simulink model "DC_AC"  (R2023a)
settings: Solver=VariableStepAuto  StartTime=0.0  StopTime=1.5  MaxStep=1e-4  RelTol=1e-3
libraries: spsMosfetLib x32, spsSeriesRLCBranchLib x29, simulink x25, spsCurrentMeasurementLib x11, spsVoltageMeasurementLib x9, spsDCVoltageSourceLib x8, spsIdealSwitchLib x5, spsDiodeLib x1, spspowerguiLib x1
(part 2 of 2)

== matlab function DC_AC/MATLAB Function ==
  data: flag input; Q14 output; compare_data input; Q23 output; u input
function [Q14,Q23]= fcn(flag, compare_data, u)

if flag == 1 %说明在正半周
    if u > compare_data %Q14导通
        Q14 = 1;        %在高电平阶段
        Q23 = 0;
    else
        Q14 = 0;
        Q23 = 0;
    end
else      %说明在负半周
    if u > compare_data
        Q23 = 1;
        Q14 = 0;
    else
        Q23 = 0;
        Q14 = 0;
    end
end

== matlab function DC_AC/Cϕx_Calculation1 ==
  data: x_Matrix input; y output; Phi input; c_Matrix input
function y = fcn(x_Matrix,Phi,c_Matrix)
a = x_Matrix;
b = Phi;
c = transpose(c_Matrix);
d = c*b
y = c*b*a;

== matlab function DC_AC/Distrubance_Calculation2 ==
  data: u input; D1_K_1 output; D1_K_2 output; D2_K_1 output; D2_K_2 output
function [D1_K_1,D1_K_2,D2_K_1,D2_K_2] = fcn(u)
d1_k_1 = (u(3)-u(4))/u(5)-u(2);
d2_k_1 = (u(1)-u(2)/u(5))-(u(6)*u(11)/(u(7)*u(8)))-(u(4)/(u(7)*u(8)))-(u(10)/(u(7)*u(8)))-(u(2)/(u(9)*u(8)));%d2(k-1)


D1_K_1 = d1_k_1;
D2_K_1 = d2_k_1;
D1_K_2 = u(12);
D2_K_2 = u(13);

== matlab function DC_AC/Distrubance_Calculation3 ==
  data: D1_K_1 input; C_d_Value output; D1_K_2 input; D2_K_1 input; D2_K_2 input; c input
function C_d_Value = fcn(D1_K_1, D1_K_2, D2_K_1, D2_K_2, c)
Distrubance_Matrix = [0;0;(2*D1_K_1-D1_K_2);(2*D2_K_1-D2_K_2)];
c_Matrix = transpose(c);
C_d_Value = c_Matrix*Distrubance_Matrix;

== matlab function DC_AC/Distrubance_Calculation1 ==
  data: D1_K_1 input; C_d_Value output; D1_K_2 input; D2_K_1 input; D2_K_2 input; c input
function C_d_Value = fcn(D1_K_1, D1_K_2, D2_K_1, D2_K_2, c)
Distrubance_Matrix = [0;0;(2*D1_K_1-D1_K_2);(2*D2_K_1-D2_K_2)];
c_Matrix = transpose(c);
C_d_Value = c_Matrix*Distrubance_Matrix;

== matlab function DC_AC/MATLAB Function2 ==
  data: flag input; Q14 output; compare_data input; Q23 output; u input
function [Q14,Q23]= fcn(flag, compare_data, u)

if flag == 1 %说明在正半周
    if u > compare_data %Q14导通
        Q14 = 1;        %在高电平阶段
        Q23 = 0;
    else
        Q14 = 0;
        Q23 = 0;
    end
else      %说明在负半周
    if u > compare_data
        Q23 = 1;
        Q14 = 0;
    else
        Q23 = 0;
        Q14 = 0;
    end
end

== matlab function DC_AC/MATLAB Function3 ==
  data: desert input; flag output
function flag = fcn(desert)
if desert >= 0 %如果在正半周的情况下导通Q1,Q4
    flag = 1;  %在正半周标志     
else
    flag = -1;    %在负半周标志%如果在负半周的情况下导通Q2,Q3
end

== matlab function DC_AC/MATLAB Function6 ==
  data: u input; v_o output; data input; i_l output
function [v_o,i_l]  = fcn(u, data)
if u < 0
    v_o = -u;
else
    v_o = u;
end

if data < 0
    i_l = -data;
else 
    i_l = data;
end

== matlab function DC_AC/MATLAB Function7 ==
  data: u input; Output output
function Output = fcn(u)
if u(1)<u(2)
    Output = 1;
else
    Output = 0;
end

== matlab function DC_AC/Sk_Calculation1 ==
  data: u input; Sk_Value output; x_Matrix output; c input
function [Sk_Value,x_Matrix] = fcn(u, c)
Sk = 0;
Matrix_C = transpose(c);

Matrix_x = [u(1);u(2);u(3);u(4)];

Sk = Matrix_C * Matrix_x;
Sk_Value = Sk;
x_Matrix = Matrix_x

== matlab function DC_AC/δ//ϕ_Calculation ==
  data: u input; y output
function y = fcn(u)
a = abs(u(4))+1;
b = power(a,-u(3));
Phi = u(2) + (1-u(2))*b;
Delta_Phi = u(1)/Phi;
y = Delta_Phi;

== matlab function DC_AC/e1_Calculation1 ==
  data: u input; Fact_e1 output; Last_e1 output
function [Fact_e1,Last_e1] = fcn(u)

Fact_e1 = u(1) - u(2);
Last_e1 = u(3);

== matlab function DC_AC/e2_Calculation1 ==
  data: u input; Fact_e2 output; Last_e2 output
function [Fact_e2,Last_e2] = fcn(u)
e2_last = u(6);
e2_fact = (u(1)/u(4))-(u(3)/(u(5)*u(4)))-u(2);
Fact_e2 = e2_fact;
Last_e2 = e2_last;

== matlab function DC_AC/MATLAB Function4 ==
  data: u input; v_o output; data input; i_l output
function [v_o,i_l]  = fcn(u, data)
if u < 0
    v_o = -u;
else
    v_o = u;
end

if data < 0
    i_l = -data;
else 
    i_l = data;
end

== matlab function DC_AC/MATLAB Function5 ==
  data: u input; y output
function y = fcn(u)
if u >0
    y = u;
else
    y = -u;
end

== matlab function DC_AC/u(k)_Calculation1 ==
  data: u input; u_k output; u_k_1 output
function [u_k,u_k_1] = fcn(u)
Out_put = 0;

if u(3) < 0
   Out_put = u(1)*(u(2)*u(3)+u(4)-u(5)-u(6));
end   

if u(3) > 0
   Out_put = u(1)*(u(2)*u(3)-u(4)-u(5)-u(6));
end

if u(3) == 0
    Out_put = u(1)*(u(2)*u(3)-u(5)-u(6));
end

u_k = Out_put;
u_k_1 = u(7);

== matlab function DC_AC/δ//ϕ_Calculation1 ==
  data: u input; y output
function y = fcn(u)
a = abs(u(4))+1;
b = power(a,-u(3));
Phi = u(2) + (1-u(2))*b;
Delta_Phi = u(1)/Phi;
y = Delta_Phi;

== matlab function DC_AC/(CΓ)'_Calculation2 ==
  data: u input; C_Gamma_Inv output; Phi output; c input
function [C_Gamma_Inv,Phi] = fcn(u, c)
coder.extrinsic('Phi_Gama_Calculation');  %引入外部函数eAtao_integral(用于计算eAtao的积分值)

Matrix_C = transpose(c);%调参矩阵

[D_Matrix_Phi,D_Matrix_Gamma] = Phi_Gama_Calculation(u(1),u(2),u(3),u(4),u(5),u(6));%计算离散情况下的A,B矩阵
    
C_Gamma_Inv = 0;       %使用外部函数返回的 mxArrays，必须先将它们转换为已知类型，此处将其转化为双精度标量值
Phi = [0 0 0 0;
       0 0 0 0;
       0 0 0 0;
       0 0 0 0];        
C_Gamma_Inv = inv(Matrix_C*D_Matrix_Gamma); %计算参数矩阵C和Gamma的逆
Phi = D_Matrix_Phi;

== matlab function DC_AC/Cϕx_Calculation2 ==
  data: x_Matrix input; y output; Phi input; c_Matrix input
function y = fcn(x_Matrix,Phi,c_Matrix)
a = x_Matrix;
b = Phi;
c = transpose(c_Matrix);
d = c*b
y = c*b*a;

== matlab function DC_AC/e1_Calculation ==
  data: u input; Fact_e1 output; Last_e1 output
function [Fact_e1,Last_e1] = fcn(u)

Fact_e1 = u(1) - u(2);
Last_e1 = u(3);

== matlab function DC_AC/Distrubance_Calculation4 ==
  data: u input; D1_K_1 output; D1_K_2 output; D2_K_1 output; D2_K_2 output
function [D1_K_1,D1_K_2,D2_K_1,D2_K_2] = fcn(u)
d1_k_1 = (u(3)-u(4))/u(5)-u(2);
d2_k_1 = (u(1)-u(2)/u(5))-(u(6)*u(11)/(u(7)*u(8)))-(u(4)/(u(7)*u(8)))-(u(10)/(u(7)*u(8)))-(u(2)/(u(9)*u(8)));%d2(k-1)


D1_K_1 = d1_k_1;
D2_K_1 = d2_k_1;
D1_K_2 = u(12);
D2_K_2 = u(13);

== matlab function DC_AC/Distrubance_Calculation5 ==
  data: D1_K_1 input; C_d_Value output; D1_K_2 input; D2_K_1 input; D2_K_2 input; c input
function C_d_Value = fcn(D1_K_1, D1_K_2, D2_K_1, D2_K_2, c)
Distrubance_Matrix = [0;0;(2*D1_K_1-D1_K_2);(2*D2_K_1-D2_K_2)];
c_Matrix = transpose(c);
C_d_Value = c_Matrix*Distrubance_Matrix;

== matlab function DC_AC/MATLAB Function10 ==
  data: u input; v_o output; data input; i_l output
function [v_o,i_l]  = fcn(u, data)
if u < 0
    v_o = -u;
else
    v_o = u;
end

if data < 0
    i_l = -data;
else 
    i_l = data;
end

== matlab function DC_AC/(CΓ)'_Calculation4 ==
  data: u input; C_Gamma_Inv output; Phi output; c input; D_Disturbance1_Matrix_k_1 output; D_Disturbance1_Matrix_k_2 output; D_k_1 input
function [C_Gamma_Inv,Phi,D_Disturbance1_Matrix_k_1,D_Disturbance1_Matrix_k_2] = fcn(u, c, D_k_1)
coder.extrinsic('Phi_Gama_Calculation');      %引入外部函数Phi_Gama_Calculation(用于计算Phi和Gamma矩阵)
coder.extrinsic('D_Distrbance_Calculation');  %引入外部函数Phi_Gama_Calculation(用于计算扰动矩阵)

Matrix_C = transpose(c);%调参矩阵

[D_Matrix_Phi,D_Matrix_Gamma] = Phi_Gama_Calculation(u(1),u(2),u(3),u(4),u(5),u(6));%计算离散情况下的A,B矩阵
C_Gamma_Inv = 0;       %使用外部函数返回的 mxArrays，必须先将它们转换为已知类型，此处将其转化为双精度标量值
Phi = [0 0 0 0;
       0 0 0 0;
       0 0 0 0;
       0 0 0 0];        
C_Gamma_Inv = inv(Matrix_C*D_Matrix_Gamma); %计算参数矩阵C和Gamma的逆
Phi = D_Matrix_Phi;

[D_Matrix_Phi2,D_Matrix_d] = D_Distrbance_Calculation(u(1),u(2),u(3),u(4),u(8)); %计算离散状况下的A,C矩阵
D_Disturbance1_Matrix_k_1 = [0;0;0;0];
D_Disturbance1_Matrix_k_1 = D_Matrix_d;
D_Disturbance1_Matrix_k_2 = [0;0;0;0];
D_Disturbance1_Matrix_k_2 = D_k_1;

== matlab function DC_AC/MATLAB Function8 ==
  data: flag input; Q14 output; compare_data input; Q23 output; u input
function [Q14,Q23]= fcn(flag, compare_data, u)

if flag == 1 %说明在正半周
    if u > compare_data %Q14导通
        Q14 = 1;        %在高电平阶段
        Q23 = 0;
    else
        Q14 = 0;
        Q23 = 0;
    end
else      %说明在负半周
    if u > compare_data
        Q23 = 1;
        Q14 = 0;
    else
        Q23 = 0;
        Q14 = 0;
    end
end

== matlab function DC_AC/MATLAB Function9 ==
  data: desert input; flag output
function flag = fcn(desert)
if desert >= 0 %如果在正半周的情况下导通Q1,Q4
    flag = 1;  %在正半周标志     
else
    flag = -1;    %在负半周标志%如果在负半周的情况下导通Q2,Q3
end

== matlab function DC_AC/Sk_Calculation2 ==
  data: u input; Sk_Value output; x_Matrix output; c input
function [Sk_Value,x_Matrix] = fcn(u, c)
Sk = 0;
Matrix_C = transpose(c);

Matrix_x = [u(1);u(2);u(3);u(4)];

Sk = Matrix_C * Matrix_x;
Sk_Value = Sk;
x_Matrix = Matrix_x

== matlab function DC_AC/e1_Calculation2 ==
  data: u input; Fact_e1 output; Last_e1 output
function [Fact_e1,Last_e1] = fcn(u)

Fact_e1 = u(1) - u(2);
Last_e1 = u(3);

== matlab function DC_AC/Sk_Calculation ==
  data: u input; Sk_Value output; x_Matrix output; c input
function [Sk_Value,x_Matrix] = fcn(u, c)
Sk = 0;
Matrix_C = transpose(c);

Matrix_x = [u(1);u(2);u(3);u(4)];

Sk = Matrix_C * Matrix_x;
Sk_Value = Sk;
x_Matrix = Matrix_x

== matlab function DC_AC/e2_Calculation2 ==
  data: u input; Fact_e2 output; Last_e2 output
function [Fact_e2,Last_e2] = fcn(u)
e2_last = u(6);
e2_fact = (u(1)/u(4))-(u(3)/(u(5)*u(4)))-u(2);
Fact_e2 = e2_fact;
Last_e2 = e2_last;

== matlab function DC_AC/u(k)_Calculation2 ==
  data: u input; u_k output; u_k_1 output
function [u_k,u_k_1] = fcn(u)
Out_put = 0;

if u(3) < 0
   Out_put = u(1)*(u(2)*u(3)+u(4)-u(5)-u(6));
end   

if u(3) > 0
   Out_put = u(1)*(u(2)*u(3)-u(4)-u(5)-u(6));
end

if u(3) == 0
    Out_put = u(1)*(u(2)*u(3)-u(5)-u(6));
end

u_k = Out_put;
u_k_1 = u(7);

== matlab function DC_AC/δ//ϕ_Calculation2 ==
  data: u input; y output
function y = fcn(u)
a = abs(u(4))+1;
b = power(a,-u(3));
Phi = u(2) + (1-u(2))*b;
Delta_Phi = u(1)/Phi;
y = Delta_Phi;

== matlab function DC_AC/(CΓ)'_Calculation3 ==
  data: u input; C_Gamma_Inv output; Phi output; c input; D_Disturbance1_Matrix_k_1 output; D_Disturbance1_Matrix_k_2 output; D_k_1 input
function [C_Gamma_Inv,Phi,D_Disturbance1_Matrix_k_1,D_Disturbance1_Matrix_k_2] = fcn(u, c, D_k_1)
coder.extrinsic('Phi_Gama_Calculation');      %引入外部函数Phi_Gama_Calculation(用于计算Phi和Gamma矩阵)
coder.extrinsic('D_Distrbance_Calculation');  %引入外部函数Phi_Gama_Calculation(用于计算扰动矩阵)

Matrix_C = transpose(c);%调参矩阵

[D_Matrix_Phi,D_Matrix_Gamma] = Phi_Gama_Calculation(u(1),u(2),u(3),u(4),u(5),u(6));%计算离散情况下的A,B矩阵
C_Gamma_Inv = 0;       %使用外部函数返回的 mxArrays，必须先将它们转换为已知类型，此处将其转化为双精度标量值
Phi = [0 0 0 0;
       0 0 0 0;
       0 0 0 0;
       0 0 0 0];        
C_Gamma_Inv = inv(Matrix_C*D_Matrix_Gamma); %计算参数矩阵C和Gamma的逆
Phi = D_Matrix_Phi;

[D_Matrix_Phi2,D_Matrix_d] = D_Distrbance_Calculation(u(1),u(2),u(3),u(4),u(8)); %计算离散状况下的A,C矩阵
D_Disturbance1_Matrix_k_1 = [0;0;0;0];
D_Disturbance1_Matrix_k_1 = [0;0;0;0];
D_Disturbance1_Matrix_k_2 = [0;0;0;0];
D_Disturbance1_Matrix_k_2 = [0;0;0;0];

== matlab function DC_AC/Cϕx_Calculation3 ==
  data: x_Matrix input; C_Phi_x output; Phi input; c_Matrix input
function C_Phi_x = fcn(x_Matrix,Phi,c_Matrix)
a = x_Matrix;
b = Phi;
c = transpose(c_Matrix);
d = c*b;
C_Phi_x = c*b*a;

== matlab function DC_AC/MATLAB Function12 ==
  data: u input; Output output
function Output = fcn(u)
if u(1)<u(2)
    Output = 1;
else
    Output = 0;
end

== matlab function DC_AC/Sk_Calculation3 ==
  data: u input; Sk_Value output; x_Matrix output; c input
function [Sk_Value,x_Matrix] = fcn(u, c)
Sk = 0;
Matrix_C = transpose(c);

Matrix_x = [u(1);u(2);u(3);u(4)];

Sk = Matrix_C * Matrix_x;
Sk_Value = Sk;
x_Matrix = Matrix_x;

== matlab function DC_AC/e1_Calculation3 ==
  data: u input; Fact_e1 output; Last_e1 output
function [Fact_e1,Last_e1] = fcn(u)
V_Value = u(1);
Fact_e1 = u(1) - u(2);
Last_e1 = u(3);

== matlab function DC_AC/e2_Calculation3 ==
  data: u input; Fact_e2 output; Last_e2 output; iL_C output; Vo_RC output
function [Fact_e2,Last_e2,iL_C,Vo_RC] = fcn(u)
i = u(1);
V_Output = u(3);
R_0 = u(5);
C = u(4);

iL_C = i/C;
Vo_RC = V_Output/(R_0*C);

e2_last = u(6);
e2_fact = (u(7)-u(8))/1e-5;%(i/C)-(V_Output/(R_0*C));
Fact_e2 = e2_fact;
Last_e2 = e2_last;

== matlab function DC_AC/u(k)_Calculation_2 ==
  data: u input; u_k output; u_k_1 output; Part_1 output; Part_2 output; Part_3 output; Disturbance output
function [u_k,u_k_1,Part_1,Part_2,Part_3,Disturbance] = fcn(u)
Out_put = 0;
C_Gamma_Inv = u(1);
alfa = u(2);
Sk = u(3);
Delta_Phi = u(4);
C_Phi_x = u(5);
Disturbance = 0;
Part_1 = 0;
Part_2 = 0;
Part_3 = 0;
Out_put = 0;

% if u(3) < 0
%    Out_put = u(1)*(u(2)*u(3)+u(4)-u(5)-u(6));
% end   
% 
% if u(3) > 0
%    Out_put = u(1)*(u(2)*u(3)-u(4)-u(5)-u(6));
% end
% 
% if u(3) == 0
%     Out_put = u(1)*(u(2)*u(3)-u(5)-u(6));
% end
if Sk < 0
   Out_put = C_Gamma_Inv*(alfa*Sk+Delta_Phi-C_Phi_x-Disturbance);
   Part_1 = alfa*Sk;
   Part_2 = Delta_Phi;
   Part_3 = -C_Phi_x;
end   

if Sk > 0
   Out_put = C_Gamma_Inv*(alfa*Sk-Delta_Phi-C_Phi_x-Disturbance);
   Part_1 = alfa*Sk;
   Part_2 = -Delta_Phi;
   Part_3 = -C_Phi_x;
end

if Sk == 0
   Out_put = C_Gamma_Inv*(alfa*Sk-C_Phi_x-Disturbance);
   Part_1 = alfa*Sk;
   Part_2 = 0;
   Part_3 = -C_Phi_x;
end

u_k = Out_put;
u_k_1 = u(7);

== matlab function DC_AC/e2_Calculation ==
  data: u input; Fact_e2 output; Last_e2 output
function [Fact_e2,Last_e2] = fcn(u)
e2_last = u(6);
e2_fact = (u(1)/u(4))-(u(3)/(u(5)*u(4)))-u(2);
Fact_e2 = e2_fact;
Last_e2 = e2_last;

== matlab function DC_AC/δ//ϕ_Calculation3 ==
  data: u input; y output
function y = fcn(u)
a = abs(u(4))+1;
b = power(a,-u(3));
Phi = u(2) + (1-u(2))*b;
Delta_Phi = u(1)/Phi;
y = Delta_Phi;

== matlab function DC_AC/MATLAB Function13 ==
  data: u input; v_o output; data input; i_l output
function [v_o,i_l]  = fcn(u, data)
if u < 0
    v_o = -u;
else
    v_o = u;
end

if data < 0
    i_l = -data;
else 
    i_l = data;
end

== matlab function DC_AC/MATLAB Function14 ==
  data: flag input; Q14 output; compare_data input; Q23 output; u input
function [Q14,Q23]= fcn(flag, compare_data, u)

if flag == 1 %说明在正半周
    if u > compare_data %Q14导通
        Q14 = 1;        %在高电平阶段
        Q23 = 0;
    else
        Q14 = 0;
        Q23 = 0;
    end
else      %说明在负半周
    if u > compare_data
        Q23 = 1;
        Q14 = 0;
    else
        Q23 = 0;
        Q14 = 0;
    end
end

== matlab function DC_AC/MATLAB Function15 ==
  data: desert input; flag output
function flag = fcn(desert)
if desert >= 0 %如果在正半周的情况下导通Q1,Q4
    flag = 1;  %在正半周标志     
else
    flag = -1;    %在负半周标志%如果在负半周的情况下导通Q2,Q3
end

== matlab function DC_AC/Cϕx_Calculation4 ==
  data: x_Matrix input; C_Phi_x output; Phi input; c_Matrix input
function C_Phi_x = fcn(x_Matrix,Phi,c_Matrix)
a = x_Matrix;
b = Phi;
c = transpose(c_Matrix);
d = c*b;
C_Phi_x = c*b*a;

== matlab function DC_AC/e1_Calculation4 ==
  data: u input; y output
function y = fcn(u)

y = (u(1) - u(2));

== matlab function DC_AC/e2_Calculation4 ==
  data: u input; y output
function y = fcn(u)

y = (u(1)/u(5))-(u(3)/(u(4)*u(5)))-u(2);

== matlab function DC_AC/u_Calculation ==
  data: u input; y output
function y = fcn(u)
L = u(9);
C = u(8);
h = u(11);   %仿真周期
E_0 = u(10);   %输入测电压
R_0 = u(7);   %理论电阻值
C_1 = u(12)   ;   %滑模面参数C_1
Out_Put = 0;
%%第一项参数P_1计算%%
P_1 = -(L*C)/(h*E_0);
%%第一项参数P_2计算%%
P_2 = C_1 * u(5);
%%第一项参数P_3计算%%
P_3 = h * (u(5)+u(2))/(L*C);
%%第一项参数P_4计算%%
P_4 = h * u(4);
%%第一项参数P_5计算%%
P_5 = (h*C_1 + 1)*u(6);
%%第一项参数P_6计算%%
P_6 = h*(u(6)-u(3))/(R_0 * C);

Out_Put = P_1*(P_2-P_3-P_4+P_5-P_6-u(1));

y = Out_Put;

== matlab function DC_AC/MATLAB Function17 ==
  data: u input; y output
function y = fcn(u)
if u >0
    y = u;
else
    y = -u;
end

== matlab function DC_AC/MATLAB Function18 ==
  data: flag input; Q14 output; compare_data input; Q23 output; u input
function [Q14,Q23]= fcn(flag, compare_data, u)

if flag == 1 %说明在正半周
    if u > compare_data %Q14导通
        Q14 = 1;        %在高电平阶段
        Q23 = 0;
    else
        Q14 = 0;
        Q23 = 0;
    end
else      %说明在负半周
    if u > compare_data
        Q23 = 1;
        Q14 = 0;
    else
        Q23 = 0;
        Q14 = 0;
    end
end

== matlab function DC_AC/Cϕx_Calculation ==
  data: x_Matrix input; y output; Phi input; c_Matrix input
function y = fcn(x_Matrix,Phi,c_Matrix)
a = x_Matrix;
b = Phi;
c = transpose(c_Matrix);
d = c*b
y = c*b*a;

== matlab function DC_AC/MATLAB Function19 ==
  data: desert input; flag output
function flag = fcn(desert)
if desert >= 0 %如果在正半周的情况下导通Q1,Q4
    flag = 1;  %在正半周标志     
else
    flag = -1;    %在负半周标志%如果在负半周的情况下导通Q2,Q3
end

== matlab function DC_AC/Distrubance_Calculation6 ==
  data: u input; D1_K_1 output; D1_K_2 output; D2_K_1 output; D2_K_2 output; Real_R_Value output; Real_E_Value output
function [D1_K_1,D1_K_2,D2_K_1,D2_K_2,Real_R_Value,Real_E_Value] = fcn(u)
e1k = u(3);
e1k_1 = u(4);
e2k = u(1);
e2k_1 = u(2);
h = u(5);
E_0 = u(6);
u_c = u(14)/u(15);
L = u(7);
C = u(8);
R_0 = u(9);
V_Output = u(14);
V_r = u(10);


d1_k_1 = ((e1k-e1k_1)/h)-e2k_1;     %检查正确
d2_k_1 = ((e2k-e2k_1)/h)-((E_0*u_c)/(L*C))-(e1k_1/(L*C))-(V_r/(L*C))-(e2k_1/(R_0*C));%d2(k-1)



%计算实际的负载R值%
d1 = d1_k_1;
Real_R = V_Output/((V_Output/R_0)-(C*d1));

%计算实际的电源电压值%
d2 = d2_k_1;
% a = (C*L*d2)/u_k_1;
% b = L/(R_0*u_k_1);
% c = V_Output/(Real_R*C);
% d = V_Output/(R_0*C);
% e = b*(c-d);
% Real_E_Value = a-e+u_k_1 * E_0;

Real_E_Value = ((C*L*d2)/u_c)-(L/(R_0*u_c))*((V_Output/(Real_R*C))-(V_Output/(R_0*C)))+(E_0/u_c);



D1_K_1 = d1_k_1;
D2_K_1 = d2_k_1;
D1_K_2 = u(12);
D2_K_2 = u(13);
Real_R_Value =Real_R;%实际的电阻值

== matlab function DC_AC/Distrubance_Calculation7 ==
  data: D1_K_1 input; C_d_Value output; D1_K_2 input; c input
function C_d_Value = fcn(D1_K_1, D1_K_2, c)
Distrubance_Matrix = 2*D1_K_1-D1_K_2;
c_Matrix = transpose(c);
C_d_Value = c_Matrix*Distrubance_Matrix;

== matlab function DC_AC/MATLAB Function11 ==
  data: compare input; Q14 output; Q23 output; u_k input; expect input
function [Q14,Q23]= fcn(compare, u_k, expect)

if expect >= 0 %如果在正半周的情况下导通Q1,Q4
    if compare<u_k
        Q14 = 1;
        Q23 = 0;
    else
        Q14 = 0;
        Q23 = 0;
    end  

else           %如果在正半周的情况下导通Q2,Q3
    if compare<u_k
        Q14 = 1;
        Q23 = 0;
    else
        Q14 = 0;
        Q23 = 0;
    end  
end

% if u_k > expect
%     Q14 = 1
% else
%     Q14 = 0
% end
% 
% Q23 = 0;
    % if compare<u_k
    %     Q14 = 1;
    %     Q23 = 0;
    % else
    %     Q14 = 0;
    %     Q23 = 0;
    % end

== matlab function DC_AC/Sk_Calculation4 ==
  data: u input; Sk_Value output; x_Matrix output; c input
function [Sk_Value,x_Matrix] = fcn(u, c)
Sk = 0;
Matrix_C = transpose(c);

Matrix_x = [u(1);u(2);u(3);u(4)];

Sk = Matrix_C * Matrix_x;
Sk_Value = Sk;
x_Matrix = Matrix_x;

== matlab function DC_AC/e1_Calculation5 ==
  data: u input; Fact_e1 output; Last_e1 output
function [Fact_e1,Last_e1] = fcn(u)
V_Value = u(1);
Fact_e1 = u(1) - u(2);
Last_e1 = u(3);

== matlab function DC_AC/e2_Calculation5 ==
  data: u input; Fact_e2 output; Last_e2 output; iL_C output; Vo_RC output
function [Fact_e2,Last_e2,iL_C,Vo_RC] = fcn(u)
i = u(1);
V_Output = u(3);
R_0 = u(5);
C = u(4);

iL_C = i/C;
Vo_RC = V_Output/(R_0*C);

e2_last = u(6);
e2_fact = (u(7)-u(8))/1e-5;%(i/C)-(V_Output/(R_0*C));
Fact_e2 = e2_fact;
Last_e2 = e2_last;

== matlab function DC_AC/u(k)_Calculation3 ==
  data: u input; u_k output; u_k_1 output; Part_1 output; Part_2 output; Part_3 output
function [u_k,u_k_1,Part_1,Part_2,Part_3] = fcn(u)
Out_put = 0;
C_Gamma_Inv = u(1);
alfa = u(2);
Sk = u(3);
Delta_Phi = u(4);
C_Phi_x = u(5);
Disturbance = u(6);
Part_1 = 0;
Part_2 = 0;
Part_3 = 0;
Out_put = 0;

% if u(3) < 0
%    Out_put = u(1)*(u(2)*u(3)+u(4)-u(5)-u(6));
% end   
% 
% if u(3) > 0
%    Out_put = u(1)*(u(2)*u(3)-u(4)-u(5)-u(6));
% end
% 
% if u(3) == 0
%     Out_put = u(1)*(u(2)*u(3)-u(5)-u(6));
% end
if Sk < 0
   Out_put = C_Gamma_Inv*(alfa*Sk+Delta_Phi-C_Phi_x-Disturbance);
   Part_1 = alfa*Sk;
   Part_2 = Delta_Phi;
   Part_3 = -C_Phi_x;
end   

if Sk > 0
   Out_put = C_Gamma_Inv*(alfa*Sk-Delta_Phi-C_Phi_x-Disturbance);
   Part_1 = alfa*Sk;
   Part_2 = -Delta_Phi;
   Part_3 = -C_Phi_x;
end

if Sk == 0
   Out_put = C_Gamma_Inv*(alfa*Sk-C_Phi_x-Disturbance);
   Part_1 = alfa*Sk;
   Part_2 = 0;
   Part_3 = -C_Phi_x;
end

u_k = Out_put;
u_k_1 = u(7);

== matlab function DC_AC/δ//ϕ_Calculation4 ==
  data: u input; y output
function y = fcn(u)
a = abs(u(4))+1;
b = power(a,-u(3));
Phi = u(2) + (1-u(2))*b;
Delta_Phi = u(1)/Phi;
y = Delta_Phi;

== matlab function DC_AC/(CΓ)'_Calculation5 ==
  data: u input; C_Gamma_Inv output; Phi output; c input; D_Disturbance1_Matrix_k_1 output; D_Disturbance1_Matrix_k_2 output; D_k_1 input
function [C_Gamma_Inv,Phi,D_Disturbance1_Matrix_k_1,D_Disturbance1_Matrix_k_2] = fcn(u, c, D_k_1)
coder.extrinsic('Phi_Gama_Calculation');      %引入外部函数Phi_Gama_Calculation(用于计算Phi和Gamma矩阵)
coder.extrinsic('D_Distrbance_Calculation');  %引入外部函数Phi_Gama_Calculation(用于计算扰动矩阵)

Matrix_C = transpose(c);%调参矩阵

[D_Matrix_Phi,D_Matrix_Gamma] = Phi_Gama_Calculation(u(1),u(2),u(3),u(4),u(5),u(6));%计算离散情况下的A,B矩阵
C_Gamma_Inv = 0;       %使用外部函数返回的 mxArrays，必须先将它们转换为已知类型，此处将其转化为双精度标量值
Phi = [0 0 0 0;
       0 0 0 0;
       0 0 0 0;
       0 0 0 0];        
C_Gamma_Inv = inv(Matrix_C*D_Matrix_Gamma); %计算参数矩阵C和Gamma的逆
Phi = D_Matrix_Phi;

[D_Matrix_Phi2,D_Matrix_d] = D_Distrbance_Calculation(u(1),u(2),u(3),u(4),u(8)); %计算离散状况下的A,C矩阵
D_Disturbance1_Matrix_k_1 = [0;0;0;0];
D_Disturbance1_Matrix_k_1 = [0;0;0;0];
D_Disturbance1_Matrix_k_2 = [0;0;0;0];
D_Disturbance1_Matrix_k_2 = [0;0;0;0];

== matlab function DC_AC/Distrubance_Calculation ==
  data: u input; D1_K_1 output; D1_K_2 output; D2_K_1 output; D2_K_2 output
function [D1_K_1,D1_K_2,D2_K_1,D2_K_2] = fcn(u)
d1_k_1 = (u(3)-u(4))/u(5)-u(2);
d2_k_1 = (u(1)-u(2)/u(5))-(u(6)*u(11)/(u(7)*u(8)))-(u(4)/(u(7)*u(8)))-(u(10)/(u(7)*u(8)))-(u(2)/(u(9)*u(8)));%d2(k-1)


D1_K_1 = d1_k_1;
D2_K_1 = d2_k_1;
D1_K_2 = u(12);
D2_K_2 = u(13);

== matlab function DC_AC/Cϕx_Calculation5 ==
  data: x_Matrix input; C_Phi_x output; Phi input; c_Matrix input
function C_Phi_x = fcn(x_Matrix,Phi,c_Matrix)
a = x_Matrix;
b = Phi;
c = transpose(c_Matrix);
d = c*b;
C_Phi_x = c*b*a;

== matlab function DC_AC/MATLAB Function21 ==
  data: u input; v_o output; data input; i_l output
function [v_o,i_l]  = fcn(u, data)
if u < 0
    v_o = -u;
else
    v_o = u;
end

if data < 0
    i_l = -data;
else 
    i_l = data;
end

== matlab function DC_AC/MATLAB Function16 ==
  data: u input; Output output
function Output = fcn(u)
if u(1)<u(2)
    Output = 1;
else
    Output = 0;
end

== matlab function DC_AC/MATLAB Function20 ==
  data: u input; v_o output; data input; i_l output
function [v_o,i_l]  = fcn(u, data)
if u < 0
    v_o = -u;
else
    v_o = u;
end

if data < 0
    i_l = -data;
else 
    i_l = data;
end

== matlab function DC_AC/MATLAB Function22 ==
  data: flag input; Q14 output; compare_data input; Q23 output; u input
function [Q14,Q23]= fcn(flag, compare_data, u)

if flag == 1 %说明在正半周
    if u > compare_data %Q14导通
        Q14 = 1;        %在高电平阶段
        Q23 = 0;
    else
        Q14 = 0;
        Q23 = 0;
    end
else      %说明在负半周
    if u > compare_data
        Q23 = 1;
        Q14 = 0;
    else
        Q23 = 0;
        Q14 = 0;
    end
end

== matlab function DC_AC/MATLAB Function23 ==
  data: desert input; flag output
function flag = fcn(desert)
if desert >= 0 %如果在正半周的情况下导通Q1,Q4
    flag = 1;  %在正半周标志     
else
    flag = -1;    %在负半周标志%如果在负半周的情况下导通Q2,Q3
end

== matlab function DC_AC/MATLAB Function24 ==
  data: u input; y output
function y = fcn(u)
if u >0
    y = u;
else
    y = -u;
end

== matlab function DC_AC/Sk_Calculation5 ==
  data: u input; Sk_Value output; x_Matrix output; c input
function [Sk_Value,x_Matrix] = fcn(u, c)
Sk = 0;
Matrix_C = transpose(c);

Matrix_x = [u(1);u(2);u(3);u(4)];

Sk = Matrix_C * Matrix_x;
Sk_Value = Sk;
x_Matrix = Matrix_x;

== matlab function DC_AC/e1_Calculation6 ==
  data: u input; Fact_e1 output; Last_e1 output
function [Fact_e1,Last_e1] = fcn(u)
V_Value = u(1);
Fact_e1 = u(1) - u(2);
Last_e1 = u(3);

== matlab function DC_AC/e2_Calculation6 ==
  data: u input; Fact_e2 output; Last_e2 output; iL_C output; Vo_RC output
function [Fact_e2,Last_e2,iL_C,Vo_RC] = fcn(u)
i = u(1);
V_Output = u(3);
R_0 = u(5);
C = u(4);

iL_C = i/C;
Vo_RC = V_Output/(R_0*C);

e2_last = u(6);
e2_fact = (u(7)-u(8))/1e-5;%(i/C)-(V_Output/(R_0*C));
Fact_e2 = e2_fact;
Last_e2 = e2_last;

== matlab function DC_AC/u(k)_Calculation_1 ==
  data: u input; u_k output; u_k_1 output; Part_1 output; Part_2 output; Part_3 output; Disturbance output
function [u_k,u_k_1,Part_1,Part_2,Part_3,Disturbance] = fcn(u)
Out_put = 0;
C_Gamma_Inv = u(1);
alfa = u(2);
Sk = u(3);
Delta_Phi = u(4);
C_Phi_x = u(5);
Disturbance = 0;
Part_1 = 0;
Part_2 = 0;
Part_3 = 0;
Out_put = 0;

% if u(3) < 0
%    Out_put = u(1)*(u(2)*u(3)+u(4)-u(5)-u(6));
% end   
% 
% if u(3) > 0
%    Out_put = u(1)*(u(2)*u(3)-u(4)-u(5)-u(6));
% end
% 
% if u(3) == 0
%     Out_put = u(1)*(u(2)*u(3)-u(5)-u(6));
% end
if Sk < 0
   Out_put = C_Gamma_Inv*(alfa*Sk+Delta_Phi-C_Phi_x-Disturbance);
   Part_1 = alfa*Sk;
   Part_2 = Delta_Phi;
   Part_3 = -C_Phi_x;
end   

if Sk > 0
   Out_put = C_Gamma_Inv*(alfa*Sk-Delta_Phi-C_Phi_x-Disturbance);
   Part_1 = alfa*Sk;
   Part_2 = -Delta_Phi;
   Part_3 = -C_Phi_x;
end

if Sk == 0
   Out_put = C_Gamma_Inv*(alfa*Sk-C_Phi_x-Disturbance);
   Part_1 = alfa*Sk;
   Part_2 = 0;
   Part_3 = -C_Phi_x;
end

u_k = Out_put;
u_k_1 = u(7);

== matlab function DC_AC/(CΓ)'_Calculation ==
  data: u input; C_Gamma_Inv output; Phi output; c input
function [C_Gamma_Inv,Phi] = fcn(u, c)
coder.extrinsic('Phi_Gama_Calculation');  %引入外部函数eAtao_integral(用于计算eAtao的积分值)

Matrix_C = transpose(c);%调参矩阵

[D_Matrix_Phi,D_Matrix_Gamma] = Phi_Gama_Calculation(u(1),u(2),u(3),u(4),u(5),u(6));%计算离散情况下的A,B矩阵
    
C_Gamma_Inv = 0;       %使用外部函数返回的 mxArrays，必须先将它们转换为已知类型，此处将其转化为双精度标量值
Phi = [0 0 0 0;
       0 0 0 0;
       0 0 0 0;
       0 0 0 0];        
C_Gamma_Inv = inv(Matrix_C*D_Matrix_Gamma); %计算参数矩阵C和Gamma的逆
Phi = D_Matrix_Phi;

== matlab function DC_AC/δ//ϕ_Calculation5 ==
  data: u input; y output
function y = fcn(u)
a = abs(u(4))+1;
b = power(a,-u(3));
Phi = u(2) + (1-u(2))*b;
Delta_Phi = u(1)/Phi;
y = Delta_Phi;

== matlab function DC_AC/MATLAB Function25 ==
  data: flag input; Q14 output; compare_data input; Q23 output; u input
function [Q14,Q23]= fcn(flag, compare_data, u)

if flag == 1 %说明在正半周
    if u > compare_data %Q14导通
        Q14 = 1;        %在高电平阶段
        Q23 = 0;
    else
        Q14 = 0;
        Q23 = 0;
    end
else      %说明在负半周
    if u > compare_data
        Q23 = 1;
        Q14 = 0;
    else
        Q23 = 0;
        Q14 = 0;
    end
end

== matlab function DC_AC/MATLAB Function26 ==
  data: desert input; flag output
function flag = fcn(desert)
if desert >= 0 %如果在正半周的情况下导通Q1,Q4
    flag = 1;  %在正半周标志     
else
    flag = -1;    %在负半周标志%如果在负半周的情况下导通Q2,Q3
end

== matlab function DC_AC/MATLAB Function27 ==
  data: u input; y output
function y = fcn(u)
if u >0
    y = u;
else
    y = -u;
end

== matlab function DC_AC/MATLAB Function28 ==
  data: u input; y output
function y = fcn(u)
if u<0
    y = -u;
else
    y = u;
end

== matlab function DC_AC/(CΓ)'_Calculation6 ==
  data: u input; C_Gamma_Inv output; Phi output; c input; D_Disturbance1_Matrix_k_1 output; D_Disturbance1_Matrix_k_2 output; D_k_1 input
function [C_Gamma_Inv,Phi,D_Disturbance1_Matrix_k_1,D_Disturbance1_Matrix_k_2] = fcn(u, c, D_k_1)
coder.extrinsic('Phi_Gama_Calculation');      %引入外部函数Phi_Gama_Calculation(用于计算Phi和Gamma矩阵)
coder.extrinsic('D_Distrbance_Calculation');  %引入外部函数Phi_Gama_Calculation(用于计算扰动矩阵)

Matrix_C = transpose(c);%调参矩阵

[D_Matrix_Phi,D_Matrix_Gamma] = Phi_Gama_Calculation(u(1),u(2),u(3),u(4),u(5),u(6));%计算离散情况下的A,B矩阵
C_Gamma_Inv = 0;       %使用外部函数返回的 mxArrays，必须先将它们转换为已知类型，此处将其转化为双精度标量值
Phi = [0 0 0 0;
       0 0 0 0;
       0 0 0 0;
       0 0 0 0];        
C_Gamma_Inv = inv(Matrix_C*D_Matrix_Gamma); %计算参数矩阵C和Gamma的逆
Phi = D_Matrix_Phi;

[D_Matrix_Phi2,D_Matrix_d] = D_Distrbance_Calculation(u(1),u(2),u(3),u(4),u(8)); %计算离散状况下的A,C矩阵
D_Disturbance1_Matrix_k_1 = [0;0;0;0];
D_Disturbance1_Matrix_k_1 = [0;0;0;0];
D_Disturbance1_Matrix_k_2 = [0;0;0;0];
D_Disturbance1_Matrix_k_2 = [0;0;0;0];

== matlab function DC_AC/Cϕx_Calculation6 ==
  data: x_Matrix input; C_Phi_x output; Phi input; c_Matrix input
function C_Phi_x = fcn(x_Matrix,Phi,c_Matrix)
a = x_Matrix;
b = Phi;
c = transpose(c_Matrix);
d = c*b;
C_Phi_x = c*b*a;

== matlab function DC_AC/MATLAB Function29 ==
  data: u input; Output output
function Output = fcn(u)
if u(1)<u(2)
    Output = 1;
else
    Output = 0;
end

== matlab function DC_AC/MATLAB Function30 ==
  data: u input; v_o output; data input; i_l output
function [v_o,i_l]  = fcn(u, data)
if u < 0
    v_o = -u;
else
    v_o = u;
end

if data < 0
    i_l = -data;
else 
    i_l = data;
end

== matlab function DC_AC/MATLAB Function31 ==
  data: flag input; Q14 output; compare_data input; Q23 output; u input
function [Q14,Q23]= fcn(flag, compare_data, u)

if flag == 1 %说明在正半周
    if u > compare_data %Q14导通
        Q14 = 1;        %在高电平阶段
        Q23 = 0;
    else
        Q14 = 0;
        Q23 = 0;
    end
else      %说明在负半周
    if u > compare_data
        Q23 = 1;
        Q14 = 0;
    else
        Q23 = 0;
        Q14 = 0;
    end
end

== matlab function DC_AC/MATLAB Function32 ==
  data: desert input; flag output
function flag = fcn(desert)
if desert >= 0 %如果在正半周的情况下导通Q1,Q4
    flag = 1;  %在正半周标志     
else
    flag = -1;    %在负半周标志%如果在负半周的情况下导通Q2,Q3
end

== matlab function DC_AC/u(k)_Calculation ==
  data: u input; u_k output; u_k_1 output
function [u_k,u_k_1] = fcn(u)
Out_put = 0;

if u(3) < 0
   Out_put = u(1)*(u(2)*u(3)+u(4)-u(5)-u(6));
end   

if u(3) > 0
   Out_put = u(1)*(u(2)*u(3)-u(4)-u(5)-u(6));
end

if u(3) == 0
    Out_put = u(1)*(u(2)*u(3)-u(5)-u(6));
end

u_k = Out_put;
u_k_1 = u(7);

== matlab function DC_AC/MATLAB Function33 ==
  data: u input; y output
function y = fcn(u)
if u >0
    y = u;
else
    y = -u;
end

== matlab function DC_AC/Sk_Calculation6 ==
  data: u input; Sk_Value output; x_Matrix output; c input
function [Sk_Value,x_Matrix] = fcn(u, c)
Sk = 0;
Matrix_C = transpose(c);

Matrix_x = [u(1);u(2);u(3);u(4)];

Sk = Matrix_C * Matrix_x;
Sk_Value = Sk;
x_Matrix = Matrix_x;

== matlab function DC_AC/e1_Calculation7 ==
  data: u input; Fact_e1 output; Last_e1 output
function [Fact_e1,Last_e1] = fcn(u)
V_Value = u(1);
Fact_e1 = u(1) - u(2);
Last_e1 = u(3);

== matlab function DC_AC/e2_Calculation7 ==
  data: u input; Fact_e2 output; Last_e2 output; iL_C output; Vo_RC output
function [Fact_e2,Last_e2,iL_C,Vo_RC] = fcn(u)
i = u(1);
V_Output = u(3);
R_0 = u(5);
C = u(4);

iL_C = i/C;
Vo_RC = V_Output/(R_0*C);

e2_last = u(6);
e2_fact = (u(7)-u(8))/1e-5;%(i/C)-(V_Output/(R_0*C));
Fact_e2 = e2_fact;
Last_e2 = e2_last;

== matlab function DC_AC/u(k)_Calculation_3 ==
  data: u input; u_k output; u_k_1 output; Part_1 output; Part_2 output; Part_3 output; Disturbance output
function [u_k,u_k_1,Part_1,Part_2,Part_3,Disturbance] = fcn(u)
Out_put = 0;
C_Gamma_Inv = u(1);
alfa = u(2);
Sk = u(3);
Delta_Phi = u(4);
C_Phi_x = u(5);
Disturbance = 0;
Part_1 = 0;
Part_2 = 0;
Part_3 = 0;
Out_put = 0;

% if u(3) < 0
%    Out_put = u(1)*(u(2)*u(3)+u(4)-u(5)-u(6));
% end   
% 
% if u(3) > 0
%    Out_put = u(1)*(u(2)*u(3)-u(4)-u(5)-u(6));
% end
% 
% if u(3) == 0
%     Out_put = u(1)*(u(2)*u(3)-u(5)-u(6));
% end
if Sk < 0
   Out_put = C_Gamma_Inv*(alfa*Sk+Delta_Phi-C_Phi_x-Disturbance);
   Part_1 = alfa*Sk;
   Part_2 = Delta_Phi;
   Part_3 = -C_Phi_x;
end   

if Sk > 0
   Out_put = C_Gamma_Inv*(alfa*Sk-Delta_Phi-C_Phi_x-Disturbance);
   Part_1 = alfa*Sk;
   Part_2 = -Delta_Phi;
   Part_3 = -C_Phi_x;
end

if Sk == 0
   Out_put = C_Gamma_Inv*(alfa*Sk-C_Phi_x-Disturbance);
   Part_1 = alfa*Sk;
   Part_2 = 0;
   Part_3 = -C_Phi_x;
end

u_k = Out_put;
u_k_1 = u(7);

== matlab function DC_AC/δ//ϕ_Calculation6 ==
  data: u input; y output
function y = fcn(u)
a = abs(u(4))+1;
b = power(a,-u(3));
Phi = u(2) + (1-u(2))*b;
Delta_Phi = u(1)/Phi;
y = Delta_Phi;

== matlab function DC_AC/MATLAB Function1 ==
  data: desert input; flag output
function flag = fcn(desert)
if desert >= 0 %如果在正半周的情况下导通Q1,Q4
    flag = 1;  %在正半周标志     
else
    flag = -1;    %在负半周标志%如果在负半周的情况下导通Q2,Q3
end

== matlab function DC_AC/(CΓ)'_Calculation1 ==
  data: u input; C_Gamma_Inv output; Phi output; c input
function [C_Gamma_Inv,Phi] = fcn(u, c)
coder.extrinsic('Phi_Gama_Calculation');  %引入外部函数eAtao_integral(用于计算eAtao的积分值)

Matrix_C = transpose(c);%调参矩阵

[D_Matrix_Phi,D_Matrix_Gamma] = Phi_Gama_Calculation(u(1),u(2),u(3),u(4),u(5),u(6));%计算离散情况下的A,B矩阵
    
C_Gamma_Inv = 0;       %使用外部函数返回的 mxArrays，必须先将它们转换为已知类型，此处将其转化为双精度标量值
Phi = [0 0 0 0;
       0 0 0 0;
       0 0 0 0;
       0 0 0 0];        
C_Gamma_Inv = inv(Matrix_C*D_Matrix_Gamma); %计算参数矩阵C和Gamma的逆
Phi = D_Matrix_Phi;
